simulink model "Lab11"  (R2022a)
settings: Solver=VariableStepAuto  StartTime=0.0  StopTime=50  RelTol=1e-3
model workspace (MAT data in the model file):
  L = 2
  g = 9.8
  mC = 10
  mL = 60
libraries: dspsrcs4 x1, simulink x1
settings Model: Creator=ishaan  LastModifiedBy=ishaan

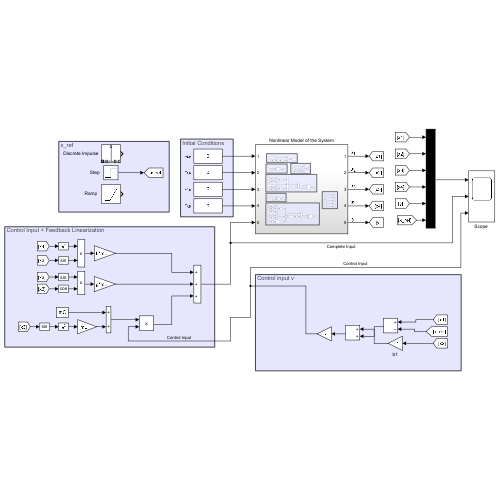
[thumbnail: Simulink's stored preview of the top-level diagram]
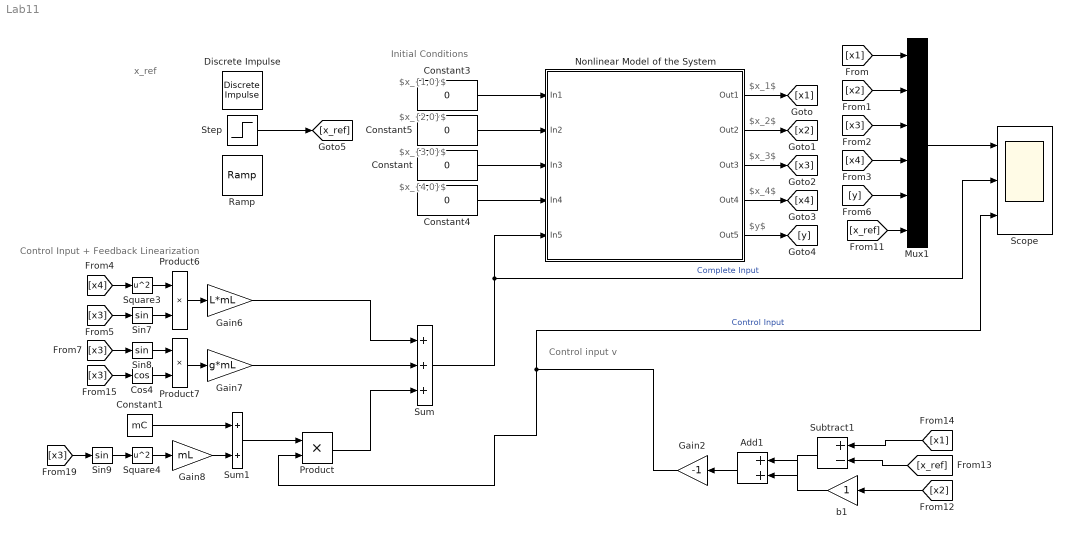
== system Lab11 ==
  note: Control input v
  note: Control Input + Feedback Linearization
  note: x_ref
  note: $x_1$
  note: $x_3$
  note: $x_{2,0}$
  note: $x_{3,0}$
  note: Initial Conditions
  note: $x_{1,0}$
  note: $x_4$
  note: $y$
  note: $x_{4,0}$
  note: $x_2$
  Add1 : Sum
  Constant{,3..5} (4 alike) : Constant  Value=0
  Constant1 : Constant  Value=mC
  Cos4 : Trigonometry  Operator=cos
  Discrete Impulse : dspsrcs4/Discrete  Impulse  Delay=0  SampleTime=1e-4  FrameSample=1  OutputFrames=off  dataType=double  isSigned=on  wordLen=16  udDataType=sfix(16)  fracBitsMode=Best precision  numFracBits=15  OutDataTypeStr=double  LastOutDataTypeStr=double
  Gain2 : Gain  Gain=-1
  Gain6 : Gain  Gain=L*mL
  Gain7 : Gain  Gain=g*mL
  Gain8 : Gain  Gain=mL
  Mux1 : Mux  Inputs=6
  Nonlinear Model of the System : Subsystem
  Product : Product
  Product6 : Product
  Product7 : Product
  "Ramp " : simulink/Sources/Ramp  slope=1  start=0  InitialOutput=0
  "Scope " : Scope  NumInputPorts=3
  Sin7 : Trigonometry
  Sin8 : Trigonometry
  Sin9 : Trigonometry
  Square3 : Math  Operator=square
  Square4 : Math  Operator=square
  "Step " : Step  Time=0  SampleTime=0
  Subtract1 : Sum  Inputs=+-
  Sum : Sum  Inputs=+++
  Sum1 : Sum
  b1 : Gain
  wires:
  Constant5/1 -> Nonlinear Model of the System/2(In2)
  Constant4/1 -> Nonlinear Model of the System/4(In4)
  Mux1/1 -> "Scope "/1
  Constant/1 -> Nonlinear Model of the System/3(In3)
  Constant3/1 -> Nonlinear Model of the System/1(In1)
  [x3] -> Sin8/1
  [x3] -> Cos4/1
  Cos4/1 -> Product7/2
  Gain7/1 -> Sum/2
  Sin8/1 -> Product7/1
  Gain8/1 -> Sum1/2
  Constant1/1 -> Sum1/1
  Sum1/1 -> Product/1
  Square4/1 -> Gain8/1
  [x3] -> Sin9/1
  Square3/1 -> Product6/1
  Sin7/1 -> Product6/2
  [x3] -> Sin7/1
  Product6/1 -> Gain6/1
  Sin9/1 -> Square4/1
  [x4] -> Square3/1
  Product7/1 -> Gain7/1
  Nonlinear Model of the System/1(Out1) -> [x1]
  Nonlinear Model of the System/5(Out5) -> [y]
  Nonlinear Model of the System/4(Out4) -> [x4]
  Nonlinear Model of the System/3(Out3) -> [x3]
  Nonlinear Model of the System/2(Out2) -> [x2]
  [y] -> Mux1/5
  [x4] -> Mux1/4
  [x3] -> Mux1/3
  [x1] -> Mux1/1
  [x2] -> Mux1/2
  Gain6/1 -> Sum/1
  Product/1 -> Sum/3
  Sum/1 -> "Scope "/2, Nonlinear Model of the System/5(In5)  "Complete Input"
  Gain2/1 -> Product/2, "Scope "/3  "Control Input"
  [x_ref] -> Mux1/6
  [x_ref] -> Subtract1/2
  b1/1 -> Add1/1
  [x1] -> Subtract1/1
  Add1/1 -> Gain2/1
  Subtract1/1 -> Add1/2
  [x2] -> b1/1
  "Step "/1 -> [x_ref]

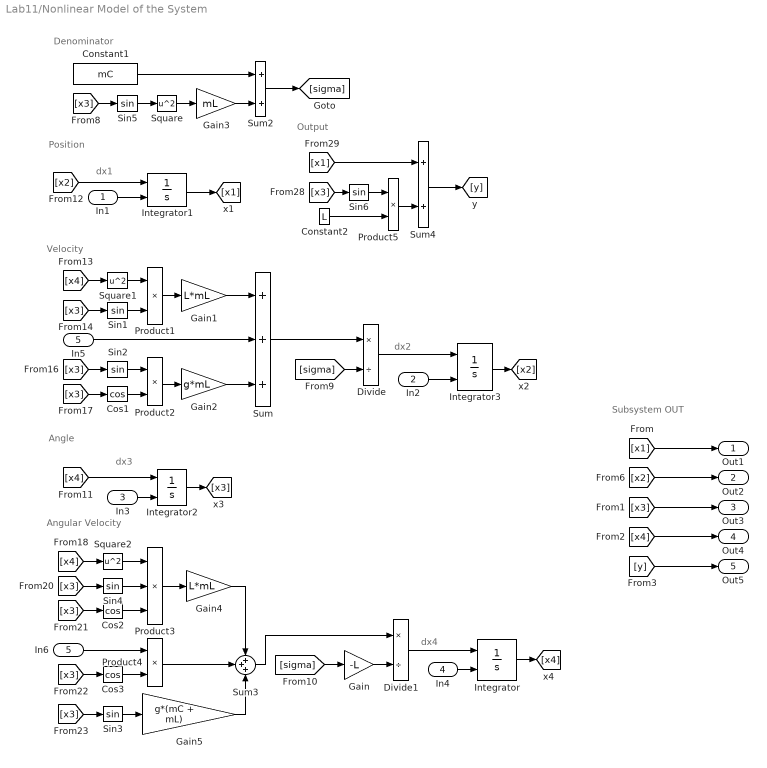
== system Lab11/Nonlinear Model of the System ==
  note: Subsystem OUT
  note: dx4
  note: dx2
  note: dx1
  note: dx3
  note: Denominator
  note: Output
  note: Position
  note: Angle
  note: Velocity
  note: Angular Velocity
  In1 : Inport
  In2 : Inport  Port=2
  In3 : Inport  Port=3
  In4 : Inport  Port=4
  In5 : Inport  Port=5
  Constant1 : Constant  Value=mC
  Constant2 : Constant  Value=L
  Cos1 : Trigonometry  Operator=cos
  Cos2 : Trigonometry  Operator=cos
  Cos3 : Trigonometry  Operator=cos
  Divide : Product  Inputs=*/
  Divide1 : Product  Inputs=*/
  Gain : Gain  Gain=-L
  Gain1 : Gain  Gain=L*mL
  Gain2 : Gain  Gain=g*mL
  Gain3 : Gain  Gain=mL
  Gain4 : Gain  Gain=L*mL
  Gain5 : Gain  Gain=g*(mC + mL)
  In6 : InportShadow  Port=5
  Integrator : Integrator  InitialConditionSource=external
  Integrator1 : Integrator  InitialConditionSource=external
  Integrator2 : Integrator  InitialConditionSource=external  InitialCondition=pi+0.01  WrappedStateUpperValue=2*pi  WrappedStateLowerValue=0
  Integrator3 : Integrator  InitialConditionSource=external
  Product{1..2,4..5} (4 alike) : Product
  Product3 : Product  Inputs=3
  Sin{1..6} (6 alike) : Trigonometry
  Square : Math  Operator=square
  Square1 : Math  Operator=square
  Square2 : Math  Operator=square
  Sum : Sum  Inputs=+++
  Sum2 : Sum
  Sum3 : Sum  Inputs=+++
  Sum4 : Sum
  Out1 : Outport
  Out2 : Outport  Port=2
  Out3 : Outport  Port=3
  Out4 : Outport  Port=4
  Out5 : Outport  Port=5
  wires:
  Sum4/1 -> [y]
  [y] -> Out5/1
  [x2] -> Integrator1/1
  [x3] -> Sin2/1
  Sin1/1 -> Product1/2
  Sum2/1 -> [sigma]
  Sum3/1 -> Divide1/1
  Product2/1 -> Gain2/1
  [x3] -> Cos3/1
  [x2] -> Out2/1
  Gain3/1 -> Sum2/2
  Divide1/1 -> Integrator/1
  [x3] -> Sin4/1
  In1/1 -> Integrator1/2
  Gain5/1 -> Sum3/3
  [sigma] -> Divide/2
  Product5/1 -> Sum4/2
  Constant2/1 -> Product5/2
  Square/1 -> Gain3/1
  Sin6/1 -> Product5/1
  Sin3/1 -> Gain5/1
  Integrator2/1 -> [x3]
  Cos1/1 -> Product2/2
  Gain4/1 -> Sum3/1
  [sigma] -> Gain/1
  [x4] -> Out4/1
  Square1/1 -> Product1/1
  [x3] -> Sin1/1
  Sum/1 -> Divide/1
  Product1/1 -> Gain1/1
  [x3] -> Cos2/1
  [x4] -> Square1/1
  Product3/1 -> Gain4/1
  [x3] -> Cos1/1
  [x1] -> Sum4/1
  In2/1 -> Integrator3/2
  [x3] -> Out3/1
  Sin4/1 -> Product3/2
  Sin2/1 -> Product2/1
  Gain2/1 -> Sum/3
  Gain/1 -> Divide1/2
  [x1] -> Out1/1
  Integrator/1 -> [x4]
  [x3] -> Sin6/1
  Constant1/1 -> Sum2/1
  Cos3/1 -> Product4/2
  Gain1/1 -> Sum/1
  [x4] -> Integrator2/1
  [x3] -> Sin5/1
  [x4] -> Square2/1
  In3/1 -> Integrator2/2
  In4/1 -> Integrator/2
  Cos2/1 -> Product3/3
  Square2/1 -> Product3/1
  [x3] -> Sin3/1
  Divide/1 -> Integrator3/1
  Integrator3/1 -> [x2]
  Product4/1 -> Sum3/2
  Integrator1/1 -> [x1]
  Sin5/1 -> Square/1
  In5/1 -> Sum/2
  In6/1 -> Product4/1
